simulink model "tennode_3"  (R2018b)
settings: Solver=ode3  StartTime=0.0  StopTime=5  FixedStep=Ts  RelTol=1e-3
values from neighbouring files (symbols this model uses):
  BESS_mode = 0    [load_vars.m]
  line1 = line1_length*R1    (= 0.01273)    [load_vars.m]
  line10 = line10_length*R1    (= 0.01273)    [load_vars.m]
  LINE10_en = 1    [load_vars.m]
  line11 = line11_length*R1    (= 0.01273)    [load_vars.m]
  LINE11_en = 1    [load_vars.m]
  line12 = line12_length*R1    (= 0.02546)    [load_vars.m]
  LINE12_en = 1    [load_vars.m]
  line13 = line13_length*R1    (= 0.015276)    [load_vars.m]
  LINE13_en = 1    [load_vars.m]
  line14 = line14_length*R1    (= 0.019095)    [load_vars.m]
  LINE14_en = 1    [load_vars.m]
  line15 = line15_length*R1    (= 0.014003)    [load_vars.m]
  LINE15_en = 1    [load_vars.m]
  line16 = line16_length*R1    (= 0.034371)    [load_vars.m]
  LINE16_en = 1    [load_vars.m]
  line17 = line17_length*R1    (= 0.017822)    [load_vars.m]
  LINE17_en = 1    [load_vars.m]
  LINE1_en = 1    [load_vars.m]
  line2 = line2_length*R1    (= 0.02546)    [load_vars.m]
  LINE2_en = 1    [load_vars.m]
  line3 = line3_length*R1    (= 0.015276)    [load_vars.m]
  LINE3_en = 1    [load_vars.m]
  line4 = line4_length*R1    (= 0.019095)    [load_vars.m]
  LINE4_en = 1    [load_vars.m]
  line5 = line5_length*R1    (= 0.014003)    [load_vars.m]
  LINE5_en = 1    [load_vars.m]
  line6 = line6_length*R1    (= 0.01273)    [load_vars.m]
  LINE6_en = 1    [load_vars.m]
  line7 = line7_length*R1    (= 0.03819)    [load_vars.m]
  LINE7_en = 1    [load_vars.m]
  line8 = line8_length*R1    (= 0.01273)    [load_vars.m]
  LINE8_en = 1    [load_vars.m]
  line9 = line9_length*R1    (= 0.01273)    [load_vars.m]
  LINE9_en = 1    [load_vars.m]
  t_contingency = 1    [load_vars.m]
  Ts = 0.0001    [load_vars.m]
  uDemand1 = 20e3    (= 20000)    [load_vars.m]
  uDemand10 = 20e3    (= 20000)    [load_vars.m]
  uDemand2 = 20e3    (= 20000)    [load_vars.m]
  uDemand3 = 20e3    (= 20000)    [load_vars.m]
  uDemand4 = 20e3    (= 20000)    [load_vars.m]
  uDemand5 = 20e3    (= 20000)    [load_vars.m]
  uDemand6 = 20e3    (= 20000)    [load_vars.m]
  uDemand7 = 20e3    (= 20000)    [load_vars.m]
  uDemand8 = 20e3    (= 20000)    [load_vars.m]
  uDemand9 = 20e3    (= 20000)    [load_vars.m]
undefined symbols (not defined in the file or in its folder): DER10_BESS_en, DER1_BESS_en, DER2_BESS_en, DER3_BESS_en, DER4_BESS_en, DER5_BESS_en, DER6_BESS_en, DER7_BESS_en, DER8_BESS_en, DER9_BESS_en, DR_capacity_1, DR_capacity_10, DR_capacity_2, DR_capacity_3, DR_capacity_4, DR_capacity_5, DR_capacity_6, DR_capacity_7, DR_capacity_8, DR_capacity_9, P_set1, P_set10, P_set2, P_set3, P_set4, P_set5, P_set6, P_set7, P_set8, P_set9, PV_capacity_1, PV_capacity_10, PV_capacity_2, PV_capacity_3, PV_capacity_4, PV_capacity_5, PV_capacity_6, PV_capacity_7, PV_capacity_8, PV_capacity_9, PV_en_1, PV_en_10, PV_en_2, PV_en_3, PV_en_4, PV_en_5, PV_en_6, PV_en_7, PV_en_8, PV_en_9
libraries: powerlib x232, simulink x66, powerlib_meascontrol x23, sps_avr x1, spsDieselMotorModel x1
(part 5 of 7)

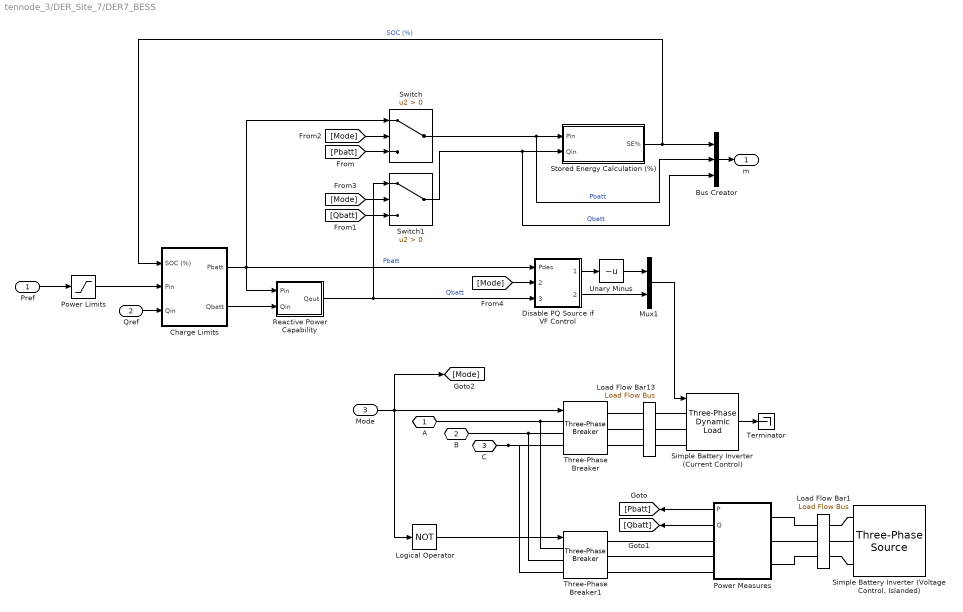
== system tennode_3/DER_Site_7/DER7_BESS ==
  Pref : Inport
  Qref : Inport  Port=2
  Mode : Inport  Port=3
  Bus Creator : BusCreator  Inputs=3
  Charge Limits : Subsystem
  Disable PQ Source if VF Control : Subsystem
  Load Flow Bar1 : powerlib/Measurements/Load Flow Bus  LConnTagsString=a|b|c  RConnTagsString=a|b|c  Phases=ABC  Connectors=on both sides  ID=5  Vbase=400/sqrt(3)  Vref=[1.0 1.0 1.0]  Vangle=[0 -120 120]  VLF=0.9823  VLFb=1.055  VLFc=0.9746  angleLF=-5.476  angleLFb=-122.5  angleLFc=116
      settings: AttributesFormatString=%<ID>  SourceProductName=Simscape Power Systems
  Load Flow Bar13 : powerlib/Measurements/Load Flow Bus  LConnTagsString=a|b|c  RConnTagsString=a|b|c  Phases=ABC  Connectors=on both sides  ID=4  Vbase=400/sqrt(3)  Vref=[1.0 1.0 1.0]  Vangle=[0 -120 120]  VLF=0.9823  VLFb=1.055  VLFc=0.9746  angleLF=-5.476  angleLFb=-122.5  angleLFc=116
      settings: AttributesFormatString=%<ID>  SourceProductName=Simscape Power Systems
  Logical Operator : Logic  Operator=NOT  AllPortsSameDT=off  OutDataTypeStr=boolean
  Mux1 : Mux  Inputs=2
  Power Limits : Saturate  UpperLimit=Pnom  LowerLimit=-Pnom
  Power Measures : Subsystem  VariantControlMode=Label  Variant=on  LabelModeActiveChoice=EMT
  Reactive Power Capability : Subsystem
  Simple Battery Inverter (Current Control) : powerlib/Elements/Three-Phase Dynamic Load  NominalVoltage=[Vn Fn]  ActiveReactivePowers=[-5000 -3.38813e-13]  PositiveSequence=[0.999844 -0.0038635]  ExternalControl=on  NpNq=[1.3 2]  TimeConstants="[0  0  0  0]"  MinimumVoltage=0.7  Tfilter=1e-2  LoadFlowParameters=[4,0,0,0,0]
      settings: SourceProductName=Simscape Electrical  SourceProductBaseCode=PS
  "Simple Battery Inverter (Voltage Control, Islanded)" : powerlib/Electrical Sources/Three-Phase Source  InternalConnection=Yg  VoltagePhases=off  Voltage=Vn  PhaseAngle=0  Voltage_phases=[25e3 25e3 25e3]/sqrt(3)  PhaseAngles_phases=[0 -120 +120]  Frequency=Fn  NonIdealSource=off  SpecifyImpedance=off  Resistance=0.8929  Inductance=16.58e-3  ShortCircuitLevel=100e6  BaseVoltage=25e3  XRratio=7  BusType=swing  Pref=10e3  Qref=0  Prefabc=[10e3, 10e3, 10e3]  Qrefabc=[0, 0, 0]  Qmin=-inf  Qmax=inf
      settings: SourceProductName=Simscape Electrical
  Stored Energy Calculation (%) : Subsystem
  Switch : Switch  Criteria=u2 > Threshold
  Switch1 : Switch  Criteria=u2 > Threshold
  Terminator : Terminator
  Three-Phase Breaker : powerlib/Elements/Three-Phase Breaker  InitialState=closed  SwitchA=on  SwitchB=on  SwitchC=on  SwitchTimes="[1/60  5/60]"  External=on  BreakerResistance=0.01  SnubberResistance=1e6  SnubberCapacitance=inf  Measurements=None
      settings: SourceProductName=Simscape Electrical
  Three-Phase Breaker1 : powerlib/Elements/Three-Phase Breaker  InitialState=open  SwitchA=on  SwitchB=on  SwitchC=on  SwitchTimes="[1/60  5/60]"  External=on  BreakerResistance=0.01  SnubberResistance=1e6  SnubberCapacitance=inf  Measurements=None
      settings: SourceProductName=Simscape Electrical
  Unary Minus : UnaryMinus
  A : PMIOPort  Side=Right
  B : PMIOPort  Port=2  Side=Right
  C : PMIOPort  Port=3  Side=Right
  m : Outport
  wires:
  Disable PQ Source if VF Control/2(Qbatt) -> Mux1/2
  Disable PQ Source if VF Control/1(Pbatt) -> Unary Minus/1
  Reactive Power Capability/1(Qout) -> Switch1/1, Disable PQ Source if VF Control/3(Qdes)  "Qbatt"
  [Mode] -> Disable PQ Source if VF Control/2(Mode)
  Charge Limits/1(Pbatt) -> Disable PQ Source if VF Control/1(Pdes), Reactive Power Capability/1(Pin), Switch/1  "Pbatt"
  [Pbatt] -> Switch/3
  [Qbatt] -> Switch1/3
  [Mode] -> Switch1/2
  [Mode] -> Switch/2
  Switch1/1 -> Stored Energy Calculation (%)/2(Qin), Bus Creator/3  "Qbatt"
  Switch/1 -> Stored Energy Calculation (%)/1(Pin), Bus Creator/2  "Pbatt"
  Power Measures/2(Q) -> [Qbatt]
  Power Measures/1(P) -> [Pbatt]
  Mode/1 -> Three-Phase Breaker/1, Logical Operator/1, [Mode]
  Logical Operator/1 -> Three-Phase Breaker1/1
  Unary Minus/1 -> Mux1/1
  Mux1/1 -> Simple Battery Inverter (Current Control)/1
  Simple Battery Inverter (Current Control)/1 -> Terminator/1
  Pref/1 -> Power Limits/1
  Bus Creator/1 -> m/1
  Stored Energy Calculation (%)/1(SE%) -> Charge Limits/1(SOC (%)), Bus Creator/1  "SOC (%)"
  Power Limits/1 -> Charge Limits/2(Pin)
  Qref/1 -> Charge Limits/3(Qin)
  Charge Limits/2(Qbatt) -> Reactive Power Capability/2(Qin)
  connections:
  Power Measures/RConn3 -- Three-Phase Breaker1/RConn3
  Power Measures/RConn2 -- Three-Phase Breaker1/RConn2
  Power Measures/RConn1 -- Three-Phase Breaker1/RConn1
  Three-Phase Breaker1/LConn1 -- A/RConn1 -- Three-Phase Breaker/LConn1
  Three-Phase Breaker1/LConn2 -- B/RConn1 -- Three-Phase Breaker/LConn2
  C/RConn1 -- Three-Phase Breaker1/LConn3 -- Three-Phase Breaker/LConn3
  Load Flow Bar13/RConn1 -- Three-Phase Breaker/RConn1
  Load Flow Bar13/RConn2 -- Three-Phase Breaker/RConn2
  Load Flow Bar13/RConn3 -- Three-Phase Breaker/RConn3
  Load Flow Bar13/LConn1 -- Simple Battery Inverter (Current Control)/LConn1
  Load Flow Bar13/LConn2 -- Simple Battery Inverter (Current Control)/LConn2
  Load Flow Bar13/LConn3 -- Simple Battery Inverter (Current Control)/LConn3
  "Simple Battery Inverter (Voltage Control, Islanded)"/RConn2 -- Load Flow Bar1/LConn2
  Load Flow Bar1/LConn3 -- "Simple Battery Inverter (Voltage Control, Islanded)"/RConn3
  Load Flow Bar1/LConn1 -- "Simple Battery Inverter (Voltage Control, Islanded)"/RConn1
  Power Measures/LConn1 -- Load Flow Bar1/RConn1
  Power Measures/LConn2 -- Load Flow Bar1/RConn2
  Power Measures/LConn3 -- Load Flow Bar1/RConn3

== system tennode_3/DER_Site_7/DER7_PV  ==
  P : Inport
  Bus Selector : BusSelector  OutputSignals=Active power P (W)
  Constant11 : Constant  Value=0
  Mux1 : Mux  Inputs=2
  Simple Solar Inverter : powerlib/Elements/Three-Phase Dynamic Load  NominalVoltage=[Vn Fn]  ActiveReactivePowers=[-4000 -3.38813e-13]  PositiveSequence=[0.999844 -0.0038635]  ExternalControl=on  NpNq=[1.3 2]  TimeConstants="[0  0  0  0]"  MinimumVoltage=0.7  Tfilter=1e-2  LoadFlowParameters=[4,0,0,0,0]
      settings: SourceProductName=Simscape Electrical  SourceProductBaseCode=PS
  Unary Minus : UnaryMinus
  Unary Minus1 : UnaryMinus
  A : PMIOPort  Side=Right
  B : PMIOPort  Port=2  Side=Right
  C : PMIOPort  Port=3  Side=Right
  m : Outport
  wires:
  P/1 -> Unary Minus/1
  Unary Minus/1 -> Mux1/1
  Mux1/1 -> Simple Solar Inverter/1
  Constant11/1 -> Mux1/2
  Simple Solar Inverter/1 -> Bus Selector/1
  Bus Selector/1 -> Unary Minus1/1  "<Active power P (W)>"
  Unary Minus1/1 -> m/1
  connections:
  Simple Solar Inverter/LConn2 -- B/RConn1
  Simple Solar Inverter/LConn3 -- C/RConn1
  Simple Solar Inverter/LConn1 -- A/RConn1

== system tennode_3/DER_Site_7/Site Load ==
  Load : Inport
  Dynamic Load Control : Subsystem
  Simple Three-Phase Load : powerlib/Elements/Three-Phase Dynamic Load  NominalVoltage=[Vn Fn]  ActiveReactivePowers=[200000 45883.1]  PositiveSequence=[0.999844 -0.0038635]  ExternalControl=on  NpNq=[1.3 2]  TimeConstants="[0  0  0  0]"  MinimumVoltage=0.7  Tfilter=1e-2  LoadFlowParameters=[4,0,0,0,0]
      settings: SourceProductName=Simscape Electrical  SourceProductBaseCode=PS
  A : PMIOPort  Side=Right
  B : PMIOPort  Port=2  Side=Right
  C : PMIOPort  Port=3  Side=Right
  m : Outport
  wires:
  Load/1 -> Dynamic Load Control/1(P0)
  Dynamic Load Control/1(PQ) -> Simple Three-Phase Load/1
  Simple Three-Phase Load/1 -> m/1
  connections:
  Simple Three-Phase Load/LConn1 -- A/RConn1
  Simple Three-Phase Load/LConn3 -- C/RConn1
  Simple Three-Phase Load/LConn2 -- B/RConn1

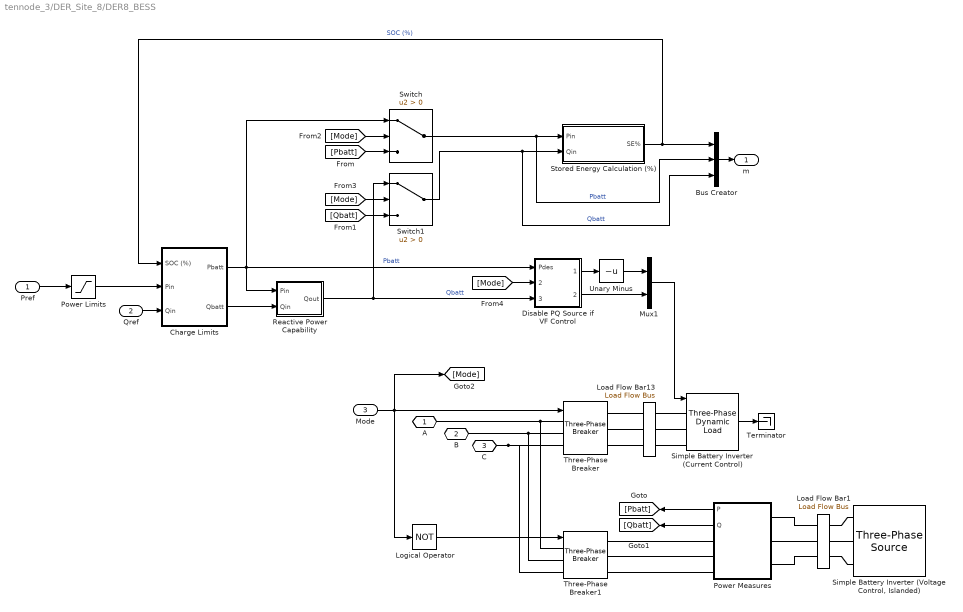
== system tennode_3/DER_Site_8/DER8_BESS ==
  Pref : Inport
  Qref : Inport  Port=2
  Mode : Inport  Port=3
  Bus Creator : BusCreator  Inputs=3
  Charge Limits : Subsystem
  Disable PQ Source if VF Control : Subsystem
  Load Flow Bar1 : powerlib/Measurements/Load Flow Bus  LConnTagsString=a|b|c  RConnTagsString=a|b|c  Phases=ABC  Connectors=on both sides  ID=5  Vbase=400/sqrt(3)  Vref=[1.0 1.0 1.0]  Vangle=[0 -120 120]  VLF=0.9823  VLFb=1.055  VLFc=0.9746  angleLF=-5.476  angleLFb=-122.5  angleLFc=116
      settings: AttributesFormatString=%<ID>  SourceProductName=Simscape Power Systems
  Load Flow Bar13 : powerlib/Measurements/Load Flow Bus  LConnTagsString=a|b|c  RConnTagsString=a|b|c  Phases=ABC  Connectors=on both sides  ID=4  Vbase=400/sqrt(3)  Vref=[1.0 1.0 1.0]  Vangle=[0 -120 120]  VLF=0.9823  VLFb=1.055  VLFc=0.9746  angleLF=-5.476  angleLFb=-122.5  angleLFc=116
      settings: AttributesFormatString=%<ID>  SourceProductName=Simscape Power Systems
  Logical Operator : Logic  Operator=NOT  AllPortsSameDT=off  OutDataTypeStr=boolean
  Mux1 : Mux  Inputs=2
  Power Limits : Saturate  UpperLimit=Pnom  LowerLimit=-Pnom
  Power Measures : Subsystem  VariantControlMode=Label  Variant=on  LabelModeActiveChoice=EMT
  Reactive Power Capability : Subsystem
  Simple Battery Inverter (Current Control) : powerlib/Elements/Three-Phase Dynamic Load  NominalVoltage=[Vn Fn]  ActiveReactivePowers=[-5000 -3.38813e-13]  PositiveSequence=[0.999844 -0.0038635]  ExternalControl=on  NpNq=[1.3 2]  TimeConstants="[0  0  0  0]"  MinimumVoltage=0.7  Tfilter=1e-2  LoadFlowParameters=[4,0,0,0,0]
      settings: SourceProductName=Simscape Electrical  SourceProductBaseCode=PS
  "Simple Battery Inverter (Voltage Control, Islanded)" : powerlib/Electrical Sources/Three-Phase Source  InternalConnection=Yg  VoltagePhases=off  Voltage=Vn  PhaseAngle=0  Voltage_phases=[25e3 25e3 25e3]/sqrt(3)  PhaseAngles_phases=[0 -120 +120]  Frequency=Fn  NonIdealSource=off  SpecifyImpedance=off  Resistance=0.8929  Inductance=16.58e-3  ShortCircuitLevel=100e6  BaseVoltage=25e3  XRratio=7  BusType=swing  Pref=10e3  Qref=0  Prefabc=[10e3, 10e3, 10e3]  Qrefabc=[0, 0, 0]  Qmin=-inf  Qmax=inf
      settings: SourceProductName=Simscape Electrical
  Stored Energy Calculation (%) : Subsystem
  Switch : Switch  Criteria=u2 > Threshold
  Switch1 : Switch  Criteria=u2 > Threshold
  Terminator : Terminator
  Three-Phase Breaker : powerlib/Elements/Three-Phase Breaker  InitialState=closed  SwitchA=on  SwitchB=on  SwitchC=on  SwitchTimes="[1/60  5/60]"  External=on  BreakerResistance=0.01  SnubberResistance=1e6  SnubberCapacitance=inf  Measurements=None
      settings: SourceProductName=Simscape Electrical
  Three-Phase Breaker1 : powerlib/Elements/Three-Phase Breaker  InitialState=open  SwitchA=on  SwitchB=on  SwitchC=on  SwitchTimes="[1/60  5/60]"  External=on  BreakerResistance=0.01  SnubberResistance=1e6  SnubberCapacitance=inf  Measurements=None
      settings: SourceProductName=Simscape Electrical
  Unary Minus : UnaryMinus
  A : PMIOPort  Side=Right
  B : PMIOPort  Port=2  Side=Right
  C : PMIOPort  Port=3  Side=Right
  m : Outport
  wires:
  Disable PQ Source if VF Control/2(Qbatt) -> Mux1/2
  Disable PQ Source if VF Control/1(Pbatt) -> Unary Minus/1
  Reactive Power Capability/1(Qout) -> Switch1/1, Disable PQ Source if VF Control/3(Qdes)  "Qbatt"
  [Mode] -> Disable PQ Source if VF Control/2(Mode)
  Charge Limits/1(Pbatt) -> Disable PQ Source if VF Control/1(Pdes), Reactive Power Capability/1(Pin), Switch/1  "Pbatt"
  [Pbatt] -> Switch/3
  [Qbatt] -> Switch1/3
  [Mode] -> Switch1/2
  [Mode] -> Switch/2
  Switch1/1 -> Stored Energy Calculation (%)/2(Qin), Bus Creator/3  "Qbatt"
  Switch/1 -> Stored Energy Calculation (%)/1(Pin), Bus Creator/2  "Pbatt"
  Power Measures/2(Q) -> [Qbatt]
  Power Measures/1(P) -> [Pbatt]
  Mode/1 -> Three-Phase Breaker/1, Logical Operator/1, [Mode]
  Logical Operator/1 -> Three-Phase Breaker1/1
  Unary Minus/1 -> Mux1/1
  Mux1/1 -> Simple Battery Inverter (Current Control)/1
  Simple Battery Inverter (Current Control)/1 -> Terminator/1
  Pref/1 -> Power Limits/1
  Bus Creator/1 -> m/1
  Stored Energy Calculation (%)/1(SE%) -> Charge Limits/1(SOC (%)), Bus Creator/1  "SOC (%)"
  Power Limits/1 -> Charge Limits/2(Pin)
  Qref/1 -> Charge Limits/3(Qin)
  Charge Limits/2(Qbatt) -> Reactive Power Capability/2(Qin)
  connections:
  Power Measures/RConn3 -- Three-Phase Breaker1/RConn3
  Power Measures/RConn2 -- Three-Phase Breaker1/RConn2
  Power Measures/RConn1 -- Three-Phase Breaker1/RConn1
  Three-Phase Breaker1/LConn1 -- A/RConn1 -- Three-Phase Breaker/LConn1
  Three-Phase Breaker1/LConn2 -- B/RConn1 -- Three-Phase Breaker/LConn2
  C/RConn1 -- Three-Phase Breaker1/LConn3 -- Three-Phase Breaker/LConn3
  Load Flow Bar13/RConn1 -- Three-Phase Breaker/RConn1
  Load Flow Bar13/RConn2 -- Three-Phase Breaker/RConn2
  Load Flow Bar13/RConn3 -- Three-Phase Breaker/RConn3
  Load Flow Bar13/LConn1 -- Simple Battery Inverter (Current Control)/LConn1
  Load Flow Bar13/LConn2 -- Simple Battery Inverter (Current Control)/LConn2
  Load Flow Bar13/LConn3 -- Simple Battery Inverter (Current Control)/LConn3
  "Simple Battery Inverter (Voltage Control, Islanded)"/RConn2 -- Load Flow Bar1/LConn2
  Load Flow Bar1/LConn3 -- "Simple Battery Inverter (Voltage Control, Islanded)"/RConn3
  Load Flow Bar1/LConn1 -- "Simple Battery Inverter (Voltage Control, Islanded)"/RConn1
  Power Measures/LConn1 -- Load Flow Bar1/RConn1
  Power Measures/LConn2 -- Load Flow Bar1/RConn2
  Power Measures/LConn3 -- Load Flow Bar1/RConn3

== system tennode_3/DER_Site_8/DER8_PV  ==
  P : Inport
  Bus Selector : BusSelector  OutputSignals=Active power P (W)
  Constant11 : Constant  Value=0
  Mux1 : Mux  Inputs=2
  Simple Solar Inverter : powerlib/Elements/Three-Phase Dynamic Load  NominalVoltage=[Vn Fn]  ActiveReactivePowers=[-4000 -3.38813e-13]  PositiveSequence=[0.999844 -0.0038635]  ExternalControl=on  NpNq=[1.3 2]  TimeConstants="[0  0  0  0]"  MinimumVoltage=0.7  Tfilter=1e-2  LoadFlowParameters=[4,0,0,0,0]
      settings: SourceProductName=Simscape Electrical  SourceProductBaseCode=PS
  Unary Minus : UnaryMinus
  Unary Minus1 : UnaryMinus
  A : PMIOPort  Side=Right
  B : PMIOPort  Port=2  Side=Right
  C : PMIOPort  Port=3  Side=Right
  m : Outport
  wires:
  P/1 -> Unary Minus/1
  Unary Minus/1 -> Mux1/1
  Mux1/1 -> Simple Solar Inverter/1
  Constant11/1 -> Mux1/2
  Simple Solar Inverter/1 -> Bus Selector/1
  Bus Selector/1 -> Unary Minus1/1  "<Active power P (W)>"
  Unary Minus1/1 -> m/1
  connections:
  Simple Solar Inverter/LConn2 -- B/RConn1
  Simple Solar Inverter/LConn3 -- C/RConn1
  Simple Solar Inverter/LConn1 -- A/RConn1

== system tennode_3/DER_Site_8/Site Load ==
  Load : Inport
  Dynamic Load Control : Subsystem
  Simple Three-Phase Load : powerlib/Elements/Three-Phase Dynamic Load  NominalVoltage=[Vn Fn]  ActiveReactivePowers=[200000 45883.1]  PositiveSequence=[0.999844 -0.0038635]  ExternalControl=on  NpNq=[1.3 2]  TimeConstants="[0  0  0  0]"  MinimumVoltage=0.7  Tfilter=1e-2  LoadFlowParameters=[4,0,0,0,0]
      settings: SourceProductName=Simscape Electrical  SourceProductBaseCode=PS
  A : PMIOPort  Side=Right
  B : PMIOPort  Port=2  Side=Right
  C : PMIOPort  Port=3  Side=Right
  m : Outport
  wires:
  Load/1 -> Dynamic Load Control/1(P0)
  Dynamic Load Control/1(PQ) -> Simple Three-Phase Load/1
  Simple Three-Phase Load/1 -> m/1
  connections:
  Simple Three-Phase Load/LConn1 -- A/RConn1
  Simple Three-Phase Load/LConn3 -- C/RConn1
  Simple Three-Phase Load/LConn2 -- B/RConn1

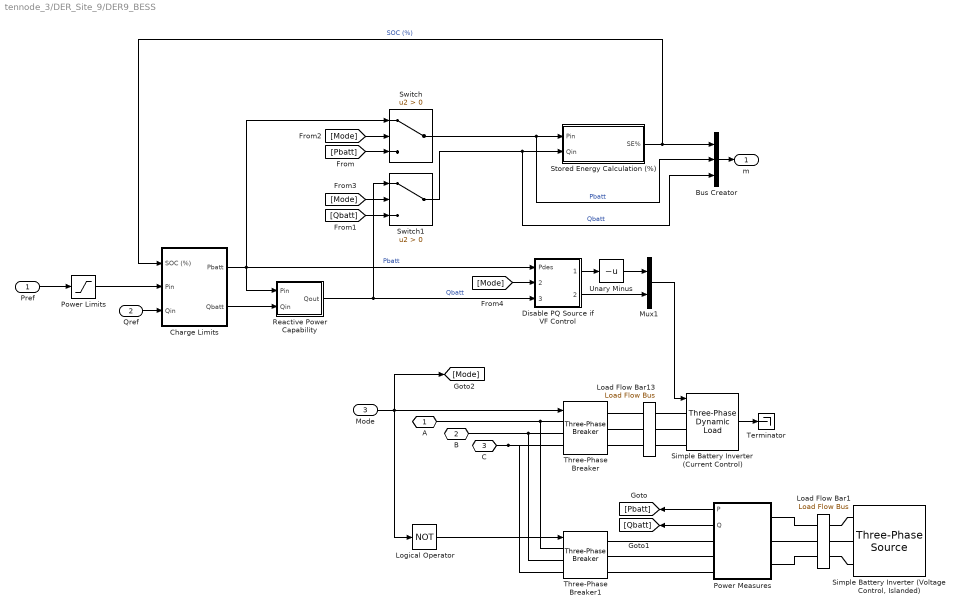
== system tennode_3/DER_Site_9/DER9_BESS ==
  Pref : Inport
  Qref : Inport  Port=2
  Mode : Inport  Port=3
  Bus Creator : BusCreator  Inputs=3
  Charge Limits : Subsystem
  Disable PQ Source if VF Control : Subsystem
  Load Flow Bar1 : powerlib/Measurements/Load Flow Bus  LConnTagsString=a|b|c  RConnTagsString=a|b|c  Phases=ABC  Connectors=on both sides  ID=5  Vbase=400/sqrt(3)  Vref=[1.0 1.0 1.0]  Vangle=[0 -120 120]  VLF=0.9823  VLFb=1.055  VLFc=0.9746  angleLF=-5.476  angleLFb=-122.5  angleLFc=116
      settings: AttributesFormatString=%<ID>  SourceProductName=Simscape Power Systems
  Load Flow Bar13 : powerlib/Measurements/Load Flow Bus  LConnTagsString=a|b|c  RConnTagsString=a|b|c  Phases=ABC  Connectors=on both sides  ID=4  Vbase=400/sqrt(3)  Vref=[1.0 1.0 1.0]  Vangle=[0 -120 120]  VLF=0.9823  VLFb=1.055  VLFc=0.9746  angleLF=-5.476  angleLFb=-122.5  angleLFc=116
      settings: AttributesFormatString=%<ID>  SourceProductName=Simscape Power Systems
  Logical Operator : Logic  Operator=NOT  AllPortsSameDT=off  OutDataTypeStr=boolean
  Mux1 : Mux  Inputs=2
  Power Limits : Saturate  UpperLimit=Pnom  LowerLimit=-Pnom
  Power Measures : Subsystem  VariantControlMode=Label  Variant=on  LabelModeActiveChoice=EMT
  Reactive Power Capability : Subsystem
  Simple Battery Inverter (Current Control) : powerlib/Elements/Three-Phase Dynamic Load  NominalVoltage=[Vn Fn]  ActiveReactivePowers=[-5000 -3.38813e-13]  PositiveSequence=[0.999844 -0.0038635]  ExternalControl=on  NpNq=[1.3 2]  TimeConstants="[0  0  0  0]"  MinimumVoltage=0.7  Tfilter=1e-2  LoadFlowParameters=[4,0,0,0,0]
      settings: SourceProductName=Simscape Electrical  SourceProductBaseCode=PS
  "Simple Battery Inverter (Voltage Control, Islanded)" : powerlib/Electrical Sources/Three-Phase Source  InternalConnection=Yg  VoltagePhases=off  Voltage=Vn  PhaseAngle=0  Voltage_phases=[25e3 25e3 25e3]/sqrt(3)  PhaseAngles_phases=[0 -120 +120]  Frequency=Fn  NonIdealSource=off  SpecifyImpedance=off  Resistance=0.8929  Inductance=16.58e-3  ShortCircuitLevel=100e6  BaseVoltage=25e3  XRratio=7  BusType=swing  Pref=10e3  Qref=0  Prefabc=[10e3, 10e3, 10e3]  Qrefabc=[0, 0, 0]  Qmin=-inf  Qmax=inf
      settings: SourceProductName=Simscape Electrical
  Stored Energy Calculation (%) : Subsystem
  Switch : Switch  Criteria=u2 > Threshold
  Switch1 : Switch  Criteria=u2 > Threshold
  Terminator : Terminator
  Three-Phase Breaker : powerlib/Elements/Three-Phase Breaker  InitialState=closed  SwitchA=on  SwitchB=on  SwitchC=on  SwitchTimes="[1/60  5/60]"  External=on  BreakerResistance=0.01  SnubberResistance=1e6  SnubberCapacitance=inf  Measurements=None
      settings: SourceProductName=Simscape Electrical
  Three-Phase Breaker1 : powerlib/Elements/Three-Phase Breaker  InitialState=open  SwitchA=on  SwitchB=on  SwitchC=on  SwitchTimes="[1/60  5/60]"  External=on  BreakerResistance=0.01  SnubberResistance=1e6  SnubberCapacitance=inf  Measurements=None
      settings: SourceProductName=Simscape Electrical
  Unary Minus : UnaryMinus
  A : PMIOPort  Side=Right
  B : PMIOPort  Port=2  Side=Right
  C : PMIOPort  Port=3  Side=Right
  m : Outport
  wires:
  Disable PQ Source if VF Control/2(Qbatt) -> Mux1/2
  Disable PQ Source if VF Control/1(Pbatt) -> Unary Minus/1
  Reactive Power Capability/1(Qout) -> Switch1/1, Disable PQ Source if VF Control/3(Qdes)  "Qbatt"
  [Mode] -> Disable PQ Source if VF Control/2(Mode)
  Charge Limits/1(Pbatt) -> Disable PQ Source if VF Control/1(Pdes), Reactive Power Capability/1(Pin), Switch/1  "Pbatt"
  [Pbatt] -> Switch/3
  [Qbatt] -> Switch1/3
  [Mode] -> Switch1/2
  [Mode] -> Switch/2
  Switch1/1 -> Stored Energy Calculation (%)/2(Qin), Bus Creator/3  "Qbatt"
  Switch/1 -> Stored Energy Calculation (%)/1(Pin), Bus Creator/2  "Pbatt"
  Power Measures/2(Q) -> [Qbatt]
  Power Measures/1(P) -> [Pbatt]
  Mode/1 -> Three-Phase Breaker/1, Logical Operator/1, [Mode]
  Logical Operator/1 -> Three-Phase Breaker1/1
  Unary Minus/1 -> Mux1/1
  Mux1/1 -> Simple Battery Inverter (Current Control)/1
  Simple Battery Inverter (Current Control)/1 -> Terminator/1
  Pref/1 -> Power Limits/1
  Bus Creator/1 -> m/1
  Stored Energy Calculation (%)/1(SE%) -> Charge Limits/1(SOC (%)), Bus Creator/1  "SOC (%)"
  Power Limits/1 -> Charge Limits/2(Pin)
  Qref/1 -> Charge Limits/3(Qin)
  Charge Limits/2(Qbatt) -> Reactive Power Capability/2(Qin)
  connections:
  Power Measures/RConn3 -- Three-Phase Breaker1/RConn3
  Power Measures/RConn2 -- Three-Phase Breaker1/RConn2
  Power Measures/RConn1 -- Three-Phase Breaker1/RConn1
  Three-Phase Breaker1/LConn1 -- A/RConn1 -- Three-Phase Breaker/LConn1
  Three-Phase Breaker1/LConn2 -- B/RConn1 -- Three-Phase Breaker/LConn2
  C/RConn1 -- Three-Phase Breaker1/LConn3 -- Three-Phase Breaker/LConn3
  Load Flow Bar13/RConn1 -- Three-Phase Breaker/RConn1
  Load Flow Bar13/RConn2 -- Three-Phase Breaker/RConn2
  Load Flow Bar13/RConn3 -- Three-Phase Breaker/RConn3
  Load Flow Bar13/LConn1 -- Simple Battery Inverter (Current Control)/LConn1
  Load Flow Bar13/LConn2 -- Simple Battery Inverter (Current Control)/LConn2
  Load Flow Bar13/LConn3 -- Simple Battery Inverter (Current Control)/LConn3
  "Simple Battery Inverter (Voltage Control, Islanded)"/RConn2 -- Load Flow Bar1/LConn2
  Load Flow Bar1/LConn3 -- "Simple Battery Inverter (Voltage Control, Islanded)"/RConn3
  Load Flow Bar1/LConn1 -- "Simple Battery Inverter (Voltage Control, Islanded)"/RConn1
  Power Measures/LConn1 -- Load Flow Bar1/RConn1
  Power Measures/LConn2 -- Load Flow Bar1/RConn2
  Power Measures/LConn3 -- Load Flow Bar1/RConn3

== system tennode_3/DER_Site_9/DER9_PV  ==
  P : Inport
  Bus Selector : BusSelector  OutputSignals=Active power P (W)
  Constant11 : Constant  Value=0
  Mux1 : Mux  Inputs=2
  Simple Solar Inverter : powerlib/Elements/Three-Phase Dynamic Load  NominalVoltage=[Vn Fn]  ActiveReactivePowers=[-4000 -3.38813e-13]  PositiveSequence=[0.999844 -0.0038635]  ExternalControl=on  NpNq=[1.3 2]  TimeConstants="[0  0  0  0]"  MinimumVoltage=0.7  Tfilter=1e-2  LoadFlowParameters=[4,0,0,0,0]
      settings: SourceProductName=Simscape Electrical  SourceProductBaseCode=PS
  Unary Minus : UnaryMinus
  Unary Minus1 : UnaryMinus
  A : PMIOPort  Side=Right
  B : PMIOPort  Port=2  Side=Right
  C : PMIOPort  Port=3  Side=Right
  m : Outport
  wires:
  P/1 -> Unary Minus/1
  Unary Minus/1 -> Mux1/1
  Mux1/1 -> Simple Solar Inverter/1
  Constant11/1 -> Mux1/2
  Simple Solar Inverter/1 -> Bus Selector/1
  Bus Selector/1 -> Unary Minus1/1  "<Active power P (W)>"
  Unary Minus1/1 -> m/1
  connections:
  Simple Solar Inverter/LConn2 -- B/RConn1
  Simple Solar Inverter/LConn3 -- C/RConn1
  Simple Solar Inverter/LConn1 -- A/RConn1

== system tennode_3/DER_Site_9/Site Load ==
  Load : Inport
  Dynamic Load Control : Subsystem
  Simple Three-Phase Load : powerlib/Elements/Three-Phase Dynamic Load  NominalVoltage=[Vn Fn]  ActiveReactivePowers=[200000 45883.1]  PositiveSequence=[0.999844 -0.0038635]  ExternalControl=on  NpNq=[1.3 2]  TimeConstants="[0  0  0  0]"  MinimumVoltage=0.7  Tfilter=1e-2  LoadFlowParameters=[4,0,0,0,0]
      settings: SourceProductName=Simscape Electrical  SourceProductBaseCode=PS
  A : PMIOPort  Side=Right
  B : PMIOPort  Port=2  Side=Right
  C : PMIOPort  Port=3  Side=Right
  m : Outport
  wires:
  Load/1 -> Dynamic Load Control/1(P0)
  Dynamic Load Control/1(PQ) -> Simple Three-Phase Load/1
  Simple Three-Phase Load/1 -> m/1
  connections:
  Simple Three-Phase Load/LConn1 -- A/RConn1
  Simple Three-Phase Load/LConn3 -- C/RConn1
  Simple Three-Phase Load/LConn2 -- B/RConn1

== system tennode_3/Frequency Measure/Diesel Generator ==
  wref (pu) : Inport
  Vref (pu) : Inport  Port=2
  AC1A Excitation System : sps_avr/AC1A Excitation System  Tr=20e-3  KaTa=[400 0.02]  VAminmax=[-14.5 14.5]  VRminmax=[-5.43 6.03]  KfTf=[0.03 1.0]  TbTc=[0 0]  KeTe=[1.0 0.80]  Ve12=[4.18 3.14]  SeVe12=[0.10 0.03]  Kd=0.38  Kc=0.20  v0=[0.99984 1.0013]  TsBlock=0
      settings: SourceProductName=Simscape Electrical  SourceProductBaseCode=PS
  Diesel Engine Governor : spsDieselMotorModel/Diesel Engine Governor  K=29  Tr=[0.01 0.02 0.2]  Ta=[0.25 0.009 0.0384]  Tlim=[0 1.1]  Td=0.024  Pm0=0.050008
  Generator Measures : Subsystem
  Ground : Ground
  Selected Measurements : Subsystem
  Shunt : powerlib/Elements/Three-Phase Parallel RLC Load  Commented=on  LConnTagsString=A|B|C  Configuration=Y (grounded)  NominalVoltage=Vn  Vabc=[1e3 1e3 1e3]  Vabcp=[1e3 1e3 1e3]  NominalFrequency=Fn  UnbalancedPower=off  ActivePower=Pn*0.05  InductivePower=0  CapacitivePower=0  Pabc=[10e3 9e3 11e3]  QLabc=[100 90 110]  QCabc=[100 90 110]  Pabcp=[10e3 9e3 11e3]  QLabcp=[100 90 110]  QCabcp=[100 90 110]  Measurements=None  LoadType=constant Z
      settings: SourceProductName=Simscape Electrical
  Synchronous Machine : powerlib/Machines/Synchronous Machine pu Standard  PresetModel=No  MechanicalLoad=Mechanical power Pm  ShowDetailedParameters=on  RotorType=Salient-pole  Units=per unit standard parameters  MeasurementBus=off  NominalParameters=[ Pn Vn Fn]  Reactances1=[ 1.81, 0.3, 0.23, 1.76, 0.65, 0.25, 0.15 ]  Reactances2="[ 1.305, 0.296, 0.252, 0.474,  0.243,  0.18 ]"  dAxisTimeConstants=Open-circuit  qAxisTimeConstants=Short-circuit  TimeConstants1="[ 4.4849  0.0681  0.1  ]"  TimeConstants2=[ 8.0, 0.03, 1.0, 0.07 ]  TimeConstants3="[  4.49  0.0681  0.0513  ]"  TimeConstants4=[ 8.0, 0.03, 0.3371, 0.0295 ]  TimeConstants5=[ 1.01, 0.053, 0.1 ]  TimeConstants6=[ 1.3201, 0.023, 1.0, 0.07 ]  TimeConstants7=[0.012 0.003 0.003]  TimeConstants8=[ 1.3201, 0.0231, 0.3371, 0.0295 ]  StatorResistance=0.003  Mechanical=[3.7 0 1 ]  PolePairs=20  InitialConditions=[0 -88.646 0.0500078 0.0500078 0.0500078 -0.0038635 -120.004 119.996 1.00126]  SetSaturation=off  Saturation=[0.6404,0.7127,0.8441,0.9214,0.9956,1.082,1.19,1.316,1.457;0.7,0.7698,0.8872,0.9466,0.9969,1.046,1.1,1.151,1.201]  LoadFlowParameters=[1,0,0,0,0]  TsPowergui=0  TsBlock=-1  IterativeModel=Trapezoidal non iterative  IterativeDiscreteModel=Trapezoidal non iterative  BusType=PQ  Pref=Pn*P0  Qref=0  Qmin=-inf  Qmax=inf  PLF=0  QLF=0
      settings: SourceProductName=Simscape Electrical
  A : PMIOPort  Side=Right
  B : PMIOPort  Port=2  Side=Right
  C : PMIOPort  Port=3  Side=Right
  m : Outport
  wires:
  wref (pu)/1 -> Diesel Engine Governor/1
  Diesel Engine Governor/1 -> Synchronous Machine/1
  AC1A Excitation System/1 -> Synchronous Machine/2
  Vref (pu)/1 -> AC1A Excitation System/1
  Synchronous Machine/1 -> Generator Measures/1(m), Selected Measurements/1(m)
  Ground/1 -> AC1A Excitation System/4
  Generator Measures/3(wm) -> Diesel Engine Governor/2
  Generator Measures/2(Vt) -> AC1A Excitation System/2
  Generator Measures/1(Ifd) -> AC1A Excitation System/3
  Selected Measurements/1(sm) -> m/1
  connections:
  Shunt/LConn1 -- Synchronous Machine/RConn1 -- A/RConn1
  Synchronous Machine/RConn3 -- Shunt/LConn3 -- C/RConn1
  Synchronous Machine/RConn2 -- Shunt/LConn2 -- B/RConn1

== system tennode_3/DER_BESS1/Charge Limits/Overcharge Check ==
  SOC (%) : Inport
  Pin : Inport  Port=2
  Qin : Inport  Port=3
  Backlash : Backlash  BacklashWidth=1e-3  InitialOutput=Initial_kWh_pc  ZeroCross=off
  Compare To Constant : simulink/Logic and Bit Operations/Compare To Constant  relop=>  const=UpChrgLim  OutDataTypeStr=boolean
  Compare To Zero : simulink/Logic and Bit Operations/Compare To Zero  relop=<=  OutDataTypeStr=boolean
  Constant : Constant  Value=0
  Constant1 : Constant  Value=0
  Logical Operator : Logic  AllPortsSameDT=off  OutDataTypeStr=boolean
  Switch : Switch  Criteria=u2 ~= 0
  Switch1 : Switch  Criteria=u2 ~= 0
  Pout : Outport
  Qout : Outport  Port=2
  wires:
  Compare To Constant/1 -> Logical Operator/1
  Logical Operator/1 -> Switch1/2, Switch/2
  Constant/1 -> Switch/1
  SOC (%)/1 -> Backlash/1
  Pin/1 -> Compare To Zero/1, Switch/3
  Switch/1 -> Pout/1
  Compare To Zero/1 -> Logical Operator/2
  Qin/1 -> Switch1/3
  Constant1/1 -> Switch1/1
  Switch1/1 -> Qout/1
  Backlash/1 -> Compare To Constant/1

== system tennode_3/DER_BESS1/Charge Limits/Undercharge Check ==
  SOC (%) : Inport
  Pin : Inport  Port=2
  Qin : Inport  Port=3
  Backlash : Backlash  BacklashWidth=1e-3  InitialOutput=Initial_kWh_pc  ZeroCross=off
  Compare To Constant1 : simulink/Logic and Bit Operations/Compare To Constant  relop=<  const=LowChrgLim  OutDataTypeStr=boolean
  Compare To Zero : simulink/Logic and Bit Operations/Compare To Zero  relop=>  OutDataTypeStr=boolean
  Constant{,1..3} (4 alike) : Constant  Value=0
  Constant4 : Constant  Value=autoRecharge
  IC : InitialCondition  Value=RechargeSOC
  Logical Operator : Logic  AllPortsSameDT=off  OutDataTypeStr=boolean
  Relay : Relay  OnSwitchValue=RechargeSOC  OffSwitchValue=LowChrgLim  OnOutputValue=0  OffOutputValue=-Precharge/100*Pnom
  Switch{,1..4} (5 alike) : Switch  Criteria=u2 ~= 0
  Pout : Outport
  Qout : Outport  Port=2
  wires:
  Compare To Zero/1 -> Logical Operator/2
  Pin/1 -> Switch/3, Compare To Zero/1
  SOC (%)/1 -> Backlash/1
  Constant/1 -> Switch/1
  Logical Operator/1 -> Switch/2, Switch1/2
  Compare To Constant1/1 -> Logical Operator/1
  Constant1/1 -> Switch1/1
  Qin/1 -> Switch1/3
  Backlash/1 -> IC/1, Compare To Constant1/1
  Switch4/1 -> Switch2/1, Switch2/2, Switch3/2
  IC/1 -> Relay/1
  Switch/1 -> Switch2/3
  Switch2/1 -> Pout/1
  Switch3/1 -> Qout/1
  Switch1/1 -> Switch3/3
  Constant2/1 -> Switch3/1
  Relay/1 -> Switch4/1
  Constant3/1 -> Switch4/3
  Constant4/1 -> Switch4/2

== system tennode_3/DER_BESS1/Power Measures/EMT ==
  "Power (3ph, Instantaneous)" : powerlib_meascontrol/Measurements/Power (3ph, Instantaneous)
      settings: SourceProductName=Simscape Electrical
  Three-Phase V-I Measurement : powerlib/Measurements/Three-Phase V-I Measurement  VoltageMeasurement=phase-to-ground  SetLabelV=off  LabelV=Vabc  Vpu=off  VpuLL=off  CurrentMeasurement=yes  SetLabelI=off  LabelI=Iabc  Ipu=off  Pbase=100e6  Vbase=500e3  OutputType=Complex  PhasorSimulation=on  PSBequivalent=0
      settings: SourceProductName=Simscape Electrical
  A : PMIOPort  Side=Left
  a : PMIOPort  Port=2  Side=Right
  B : PMIOPort  Port=3  Side=Left
  b : PMIOPort  Port=4  Side=Right
  C : PMIOPort  Port=5  Side=Left
  c : PMIOPort  Port=6  Side=Right
  P : Outport
  Q : Outport  Port=2
  wires:
  "Power (3ph, Instantaneous)"/2 -> Q/1
  "Power (3ph, Instantaneous)"/1 -> P/1
  Three-Phase V-I Measurement/1 -> "Power (3ph, Instantaneous)"/1
  Three-Phase V-I Measurement/2 -> "Power (3ph, Instantaneous)"/2
  connections:
  C/RConn1 -- Three-Phase V-I Measurement/LConn3
  c/RConn1 -- Three-Phase V-I Measurement/RConn3
  Three-Phase V-I Measurement/LConn2 -- B/RConn1
  A/RConn1 -- Three-Phase V-I Measurement/LConn1
  b/RConn1 -- Three-Phase V-I Measurement/RConn2
  Three-Phase V-I Measurement/RConn1 -- a/RConn1

== system tennode_3/DER_BESS1/Power Measures/Phasor ==
  "Power (3ph, Phasor)" : powerlib_meascontrol/Measurements/Power (3ph, Phasor)
      settings: SourceProductName=Simscape Electrical  SourceProductBaseCode=PS
  Three-Phase V-I Measurement : powerlib/Measurements/Three-Phase V-I Measurement  VoltageMeasurement=phase-to-ground  SetLabelV=off  LabelV=Vabc  Vpu=off  VpuLL=off  CurrentMeasurement=yes  SetLabelI=off  LabelI=Iabc  Ipu=off  Pbase=100e6  Vbase=500e3  OutputType=Complex  PhasorSimulation=on  PSBequivalent=0
      settings: SourceProductName=Simscape Electrical
  A : PMIOPort  Side=Left
  a : PMIOPort  Port=2  Side=Right
  B : PMIOPort  Port=3  Side=Left
  b : PMIOPort  Port=4  Side=Right
  C : PMIOPort  Port=5  Side=Left
  c : PMIOPort  Port=6  Side=Right
  P : Outport
  Q : Outport  Port=2
  wires:
  Three-Phase V-I Measurement/2 -> "Power (3ph, Phasor)"/2
  Three-Phase V-I Measurement/1 -> "Power (3ph, Phasor)"/1
  "Power (3ph, Phasor)"/1 -> P/1
  "Power (3ph, Phasor)"/2 -> Q/1
  connections:
  Three-Phase V-I Measurement/RConn1 -- a/RConn1
  b/RConn1 -- Three-Phase V-I Measurement/RConn2
  A/RConn1 -- Three-Phase V-I Measurement/LConn1
  Three-Phase V-I Measurement/LConn2 -- B/RConn1
  c/RConn1 -- Three-Phase V-I Measurement/RConn3
  C/RConn1 -- Three-Phase V-I Measurement/LConn3

== system tennode_3/DER_Site_1/DER_BESS1/Charge Limits ==
  SOC (%) : Inport
  Pin : Inport  Port=2
  Qin : Inport  Port=3
  Overcharge Check : Subsystem
  Undercharge Check : Subsystem
  Pbatt : Outport
  Qbatt : Outport  Port=2
  wires:
  Overcharge Check/2(Qout) -> Undercharge Check/3(Qin)
  Undercharge Check/1(Pout) -> Pbatt/1  "Pbatt"
  Qin/1 -> Overcharge Check/3(Qin)
  Overcharge Check/1(Pout) -> Undercharge Check/2(Pin)
  Pin/1 -> Overcharge Check/2(Pin)
  Undercharge Check/2(Qout) -> Qbatt/1
  SOC (%)/1 -> Undercharge Check/1(SOC (%)), Overcharge Check/1(SOC (%))

== system tennode_3/DER_Site_1/DER_BESS1/Disable PQ Source if VF Control ==
  Pdes : Inport
  Mode : Inport  Port=2
  Qdes : Inport  Port=3
  Constant : Constant  Value=0
  Constant1 : Constant  Value=0
  Switch2 : Switch  Criteria=u2 > Threshold
  Switch3 : Switch  Criteria=u2 > Threshold
  Pbatt : Outport
  Qbatt : Outport  Port=2
  wires:
  Qdes/1 -> Switch3/1
  Constant/1 -> Switch2/3
  Switch3/1 -> Qbatt/1
  Constant1/1 -> Switch3/3
  Switch2/1 -> Pbatt/1
  Pdes/1 -> Switch2/1
  Mode/1 -> Switch2/2, Switch3/2

== system tennode_3/DER_Site_1/DER_BESS1/Power Measures ==
  EMT : Subsystem  VariantControl=EMT
  Phasor : Subsystem  VariantControl=Phasor
  A : PMIOPort  Side=Left
  a : PMIOPort  Port=2  Side=Right
  B : PMIOPort  Port=3  Side=Left
  b : PMIOPort  Port=4  Side=Right
  C : PMIOPort  Port=5  Side=Left
  c : PMIOPort  Port=6  Side=Right
  P : Outport
  Q : Outport  Port=2

== system tennode_3/DER_Site_1/DER_BESS1/Reactive Power Capability ==
  Pin : Inport
  Qin : Inport  Port=2
  Constant : Constant  Value=Pnom
  Math Function : Math  Operator=square  SaturateOnIntegerOverflow=on
  Math Function1 : Math  Operator=square  SaturateOnIntegerOverflow=on
  Saturation Dynamic : simulink/Discontinuities/Saturation Dynamic  OutMin=[]  OutMax=[]  OutDataTypeStr=Inherit: Same as second input  OutDataType=fixdt(1, 16)  OutScaling=2^-10  DoSatur=off
  Sqrt : Sqrt  SaturateOnIntegerOverflow=on
  Sum : Sum  Inputs=-+|
  Unary Minus : UnaryMinus
  Qout : Outport
  wires:
  Qin/1 -> Saturation Dynamic/2
  Pin/1 -> Math Function1/1
  Saturation Dynamic/1 -> Qout/1
  Unary Minus/1 -> Saturation Dynamic/3
  Sum/1 -> Sqrt/1
  Constant/1 -> Math Function/1
  Math Function/1 -> Sum/2
  Math Function1/1 -> Sum/1
  Sqrt/1 -> Unary Minus/1, Saturation Dynamic/1

== system tennode_3/DER_Site_1/DER_BESS1/Stored Energy Calculation (%) ==
  Pin : Inport
  Qin : Inport  Port=2
  Charge : Gain  Gain=Efficiency/100
  Compare To Zero : simulink/Logic and Bit Operations/Compare To Zero  relop=<=  OutDataTypeStr=boolean
  Constant : Constant  Value=kWh_Rated
  Discharge : Gain  Gain=1/(Efficiency/100)
  Divide : Product  Inputs=*/
  Gain3 : Gain  Gain=1/3600/1e3
  Gain5 : Gain  Gain=-1
  Integrator : Integrator  InitialCondition=(Initial_kWh_pc/100)*kWh_Rated*3600*1e3
  Math Function1 : Math  Operator=square  SaturateOnIntegerOverflow=on
  Math Function2 : Math  Operator=square  SaturateOnIntegerOverflow=on
  Product : Product
  Sign : Signum
  Sqrt : Sqrt  SaturateOnIntegerOverflow=on
  Sum : Sum  Inputs=|++
  Switch1 : Switch  Criteria=u2 ~= 0
  Transfer Fcn : TransferFcn  Denominator=[1 1]
  to % : Gain  Gain=100
  SE% : Outport
  wires:
  Integrator/1 -> Gain3/1
  Compare To Zero/1 -> Switch1/2
  Divide/1 -> to %/1
  Charge/1 -> Switch1/1
  Constant/1 -> Divide/2
  Gain3/1 -> Divide/1
  Switch1/1 -> Gain5/1
  Transfer Fcn/1 -> Compare To Zero/1
  to %/1 -> SE%/1
  Gain5/1 -> Integrator/1
  Discharge/1 -> Switch1/3
  Product/1 -> Charge/1, Discharge/1, Transfer Fcn/1
  Pin/1 -> Sign/1, Math Function1/1
  Qin/1 -> Math Function2/1
  Math Function1/1 -> Sum/1
  Math Function2/1 -> Sum/2
  Sum/1 -> Sqrt/1
  Sqrt/1 -> Product/2
  Sign/1 -> Product/1

== system tennode_3/DER_Site_1/Site Load/Dynamic Load Control ==
  P0 : Inport
  Fcn : Fcn  Expr=sqrt(1/u(1)-1)
  Mux : Mux  Inputs=2
  Product : Product
  Summer1 : Constant  Value=PF
  PQ : Outport
  wires:
  Summer1/1 -> Fcn/1
  Fcn/1 -> Product/2
  P0/1 -> Product/1, Mux/1
  Mux/1 -> PQ/1
  Product/1 -> Mux/2  "Qo"

== system tennode_3/DER_Site_10/DER10_BESS/Charge Limits ==
  SOC (%) : Inport
  Pin : Inport  Port=2
  Qin : Inport  Port=3
  Overcharge Check : Subsystem
  Undercharge Check : Subsystem
  Pbatt : Outport
  Qbatt : Outport  Port=2
  wires:
  Overcharge Check/2(Qout) -> Undercharge Check/3(Qin)
  Undercharge Check/1(Pout) -> Pbatt/1  "Pbatt"
  Qin/1 -> Overcharge Check/3(Qin)
  Overcharge Check/1(Pout) -> Undercharge Check/2(Pin)
  Pin/1 -> Overcharge Check/2(Pin)
  Undercharge Check/2(Qout) -> Qbatt/1
  SOC (%)/1 -> Undercharge Check/1(SOC (%)), Overcharge Check/1(SOC (%))

== system tennode_3/DER_Site_10/DER10_BESS/Disable PQ Source if VF Control ==
  Pdes : Inport
  Mode : Inport  Port=2
  Qdes : Inport  Port=3
  Constant : Constant  Value=0
  Constant1 : Constant  Value=0
  Switch2 : Switch  Criteria=u2 > Threshold
  Switch3 : Switch  Criteria=u2 > Threshold
  Pbatt : Outport
  Qbatt : Outport  Port=2
  wires:
  Qdes/1 -> Switch3/1
  Constant/1 -> Switch2/3
  Switch3/1 -> Qbatt/1
  Constant1/1 -> Switch3/3
  Switch2/1 -> Pbatt/1
  Pdes/1 -> Switch2/1
  Mode/1 -> Switch2/2, Switch3/2

== system tennode_3/DER_Site_10/DER10_BESS/Power Measures ==
  EMT : Subsystem  VariantControl=EMT
  Phasor : Subsystem  VariantControl=Phasor
  A : PMIOPort  Side=Left
  a : PMIOPort  Port=2  Side=Right
  B : PMIOPort  Port=3  Side=Left
  b : PMIOPort  Port=4  Side=Right
  C : PMIOPort  Port=5  Side=Left
  c : PMIOPort  Port=6  Side=Right
  P : Outport
  Q : Outport  Port=2

== system tennode_3/DER_Site_10/DER10_BESS/Reactive Power Capability ==
  Pin : Inport
  Qin : Inport  Port=2
  Constant : Constant  Value=Pnom
  Math Function : Math  Operator=square  SaturateOnIntegerOverflow=on
  Math Function1 : Math  Operator=square  SaturateOnIntegerOverflow=on
  Saturation Dynamic : simulink/Discontinuities/Saturation Dynamic  OutMin=[]  OutMax=[]  OutDataTypeStr=Inherit: Same as second input  OutDataType=fixdt(1, 16)  OutScaling=2^-10  DoSatur=off
  Sqrt : Sqrt  SaturateOnIntegerOverflow=on
  Sum : Sum  Inputs=-+|
  Unary Minus : UnaryMinus
  Qout : Outport
  wires:
  Qin/1 -> Saturation Dynamic/2
  Pin/1 -> Math Function1/1
  Saturation Dynamic/1 -> Qout/1
  Unary Minus/1 -> Saturation Dynamic/3
  Sum/1 -> Sqrt/1
  Constant/1 -> Math Function/1
  Math Function/1 -> Sum/2
  Math Function1/1 -> Sum/1
  Sqrt/1 -> Unary Minus/1, Saturation Dynamic/1

== system tennode_3/DER_Site_10/DER10_BESS/Stored Energy Calculation (%) ==
  Pin : Inport
  Qin : Inport  Port=2
  Charge : Gain  Gain=Efficiency/100
  Compare To Zero : simulink/Logic and Bit Operations/Compare To Zero  relop=<=  OutDataTypeStr=boolean
  Constant : Constant  Value=kWh_Rated
  Discharge : Gain  Gain=1/(Efficiency/100)
  Divide : Product  Inputs=*/
  Gain3 : Gain  Gain=1/3600/1e3
  Gain5 : Gain  Gain=-1
  Integrator : Integrator  InitialCondition=(Initial_kWh_pc/100)*kWh_Rated*3600*1e3
  Math Function1 : Math  Operator=square  SaturateOnIntegerOverflow=on
  Math Function2 : Math  Operator=square  SaturateOnIntegerOverflow=on
  Product : Product
  Sign : Signum
  Sqrt : Sqrt  SaturateOnIntegerOverflow=on
  Sum : Sum  Inputs=|++
  Switch1 : Switch  Criteria=u2 ~= 0
  Transfer Fcn : TransferFcn  Denominator=[1 1]
  to % : Gain  Gain=100
  SE% : Outport
  wires:
  Integrator/1 -> Gain3/1
  Compare To Zero/1 -> Switch1/2
  Divide/1 -> to %/1
  Charge/1 -> Switch1/1
  Constant/1 -> Divide/2
  Gain3/1 -> Divide/1
  Switch1/1 -> Gain5/1
  Transfer Fcn/1 -> Compare To Zero/1
  to %/1 -> SE%/1
  Gain5/1 -> Integrator/1
  Discharge/1 -> Switch1/3
  Product/1 -> Charge/1, Discharge/1, Transfer Fcn/1
  Pin/1 -> Sign/1, Math Function1/1
  Qin/1 -> Math Function2/1
  Math Function1/1 -> Sum/1
  Math Function2/1 -> Sum/2
  Sum/1 -> Sqrt/1
  Sqrt/1 -> Product/2
  Sign/1 -> Product/1

== system tennode_3/DER_Site_10/Site Load/Dynamic Load Control ==
  P0 : Inport
  Fcn : Fcn  Expr=sqrt(1/u(1)-1)
  Mux : Mux  Inputs=2
  Product : Product
  Summer1 : Constant  Value=PF
  PQ : Outport
  wires:
  Summer1/1 -> Fcn/1
  Fcn/1 -> Product/2
  P0/1 -> Product/1, Mux/1
  Mux/1 -> PQ/1
  Product/1 -> Mux/2  "Qo"

== system tennode_3/DER_Site_2/DER2_BESS/Charge Limits ==
  SOC (%) : Inport
  Pin : Inport  Port=2
  Qin : Inport  Port=3
  Overcharge Check : Subsystem
  Undercharge Check : Subsystem
  Pbatt : Outport
  Qbatt : Outport  Port=2
  wires:
  Overcharge Check/2(Qout) -> Undercharge Check/3(Qin)
  Undercharge Check/1(Pout) -> Pbatt/1  "Pbatt"
  Qin/1 -> Overcharge Check/3(Qin)
  Overcharge Check/1(Pout) -> Undercharge Check/2(Pin)
  Pin/1 -> Overcharge Check/2(Pin)
  Undercharge Check/2(Qout) -> Qbatt/1
  SOC (%)/1 -> Undercharge Check/1(SOC (%)), Overcharge Check/1(SOC (%))

== system tennode_3/DER_Site_2/DER2_BESS/Disable PQ Source if VF Control ==
  Pdes : Inport
  Mode : Inport  Port=2
  Qdes : Inport  Port=3
  Constant : Constant  Value=0
  Constant1 : Constant  Value=0
  Switch2 : Switch  Criteria=u2 > Threshold
  Switch3 : Switch  Criteria=u2 > Threshold
  Pbatt : Outport
  Qbatt : Outport  Port=2
  wires:
  Qdes/1 -> Switch3/1
  Constant/1 -> Switch2/3
  Switch3/1 -> Qbatt/1
  Constant1/1 -> Switch3/3
  Switch2/1 -> Pbatt/1
  Pdes/1 -> Switch2/1
  Mode/1 -> Switch2/2, Switch3/2

== system tennode_3/DER_Site_2/DER2_BESS/Power Measures ==
  EMT : Subsystem  VariantControl=EMT
  Phasor : Subsystem  VariantControl=Phasor
  A : PMIOPort  Side=Left
  a : PMIOPort  Port=2  Side=Right
  B : PMIOPort  Port=3  Side=Left
  b : PMIOPort  Port=4  Side=Right
  C : PMIOPort  Port=5  Side=Left
  c : PMIOPort  Port=6  Side=Right
  P : Outport
  Q : Outport  Port=2

== system tennode_3/DER_Site_2/DER2_BESS/Reactive Power Capability ==
  Pin : Inport
  Qin : Inport  Port=2
  Constant : Constant  Value=Pnom
  Math Function : Math  Operator=square  SaturateOnIntegerOverflow=on
  Math Function1 : Math  Operator=square  SaturateOnIntegerOverflow=on
  Saturation Dynamic : simulink/Discontinuities/Saturation Dynamic  OutMin=[]  OutMax=[]  OutDataTypeStr=Inherit: Same as second input  OutDataType=fixdt(1, 16)  OutScaling=2^-10  DoSatur=off
  Sqrt : Sqrt  SaturateOnIntegerOverflow=on
  Sum : Sum  Inputs=-+|
  Unary Minus : UnaryMinus
  Qout : Outport
  wires:
  Qin/1 -> Saturation Dynamic/2
  Pin/1 -> Math Function1/1
  Saturation Dynamic/1 -> Qout/1
  Unary Minus/1 -> Saturation Dynamic/3
  Sum/1 -> Sqrt/1
  Constant/1 -> Math Function/1
  Math Function/1 -> Sum/2
  Math Function1/1 -> Sum/1
  Sqrt/1 -> Unary Minus/1, Saturation Dynamic/1

== system tennode_3/DER_Site_2/DER2_BESS/Stored Energy Calculation (%) ==
  Pin : Inport
  Qin : Inport  Port=2
  Charge : Gain  Gain=Efficiency/100
  Compare To Zero : simulink/Logic and Bit Operations/Compare To Zero  relop=<=  OutDataTypeStr=boolean
  Constant : Constant  Value=kWh_Rated
  Discharge : Gain  Gain=1/(Efficiency/100)
  Divide : Product  Inputs=*/
  Gain3 : Gain  Gain=1/3600/1e3
  Gain5 : Gain  Gain=-1
  Integrator : Integrator  InitialCondition=(Initial_kWh_pc/100)*kWh_Rated*3600*1e3
  Math Function1 : Math  Operator=square  SaturateOnIntegerOverflow=on
  Math Function2 : Math  Operator=square  SaturateOnIntegerOverflow=on
  Product : Product
  Sign : Signum
  Sqrt : Sqrt  SaturateOnIntegerOverflow=on
  Sum : Sum  Inputs=|++
  Switch1 : Switch  Criteria=u2 ~= 0
  Transfer Fcn : TransferFcn  Denominator=[1 1]
  to % : Gain  Gain=100
  SE% : Outport
  wires:
  Integrator/1 -> Gain3/1
  Compare To Zero/1 -> Switch1/2
  Divide/1 -> to %/1
  Charge/1 -> Switch1/1
  Constant/1 -> Divide/2
  Gain3/1 -> Divide/1
  Switch1/1 -> Gain5/1
  Transfer Fcn/1 -> Compare To Zero/1
  to %/1 -> SE%/1
  Gain5/1 -> Integrator/1
  Discharge/1 -> Switch1/3
  Product/1 -> Charge/1, Discharge/1, Transfer Fcn/1
  Pin/1 -> Sign/1, Math Function1/1
  Qin/1 -> Math Function2/1
  Math Function1/1 -> Sum/1
  Math Function2/1 -> Sum/2
  Sum/1 -> Sqrt/1
  Sqrt/1 -> Product/2
  Sign/1 -> Product/1

== system tennode_3/DER_Site_2/Site Load/Dynamic Load Control ==
  P0 : Inport
  Fcn : Fcn  Expr=sqrt(1/u(1)-1)
  Mux : Mux  Inputs=2
  Product : Product
  Summer1 : Constant  Value=PF
  PQ : Outport
  wires:
  Summer1/1 -> Fcn/1
  Fcn/1 -> Product/2
  P0/1 -> Product/1, Mux/1
  Mux/1 -> PQ/1
  Product/1 -> Mux/2  "Qo"

== system tennode_3/DER_Site_3/DER3_BESS/Charge Limits ==
  SOC (%) : Inport
  Pin : Inport  Port=2
  Qin : Inport  Port=3
  Overcharge Check : Subsystem
  Undercharge Check : Subsystem
  Pbatt : Outport
  Qbatt : Outport  Port=2
  wires:
  Overcharge Check/2(Qout) -> Undercharge Check/3(Qin)
  Undercharge Check/1(Pout) -> Pbatt/1  "Pbatt"
  Qin/1 -> Overcharge Check/3(Qin)
  Overcharge Check/1(Pout) -> Undercharge Check/2(Pin)
  Pin/1 -> Overcharge Check/2(Pin)
  Undercharge Check/2(Qout) -> Qbatt/1
  SOC (%)/1 -> Undercharge Check/1(SOC (%)), Overcharge Check/1(SOC (%))

== system tennode_3/DER_Site_3/DER3_BESS/Disable PQ Source if VF Control ==
  Pdes : Inport
  Mode : Inport  Port=2
  Qdes : Inport  Port=3
  Constant : Constant  Value=0
  Constant1 : Constant  Value=0
  Switch2 : Switch  Criteria=u2 > Threshold
  Switch3 : Switch  Criteria=u2 > Threshold
  Pbatt : Outport
  Qbatt : Outport  Port=2
  wires:
  Qdes/1 -> Switch3/1
  Constant/1 -> Switch2/3
  Switch3/1 -> Qbatt/1
  Constant1/1 -> Switch3/3
  Switch2/1 -> Pbatt/1
  Pdes/1 -> Switch2/1
  Mode/1 -> Switch2/2, Switch3/2

== system tennode_3/DER_Site_3/DER3_BESS/Power Measures ==
  EMT : Subsystem  VariantControl=EMT
  Phasor : Subsystem  VariantControl=Phasor
  A : PMIOPort  Side=Left
  a : PMIOPort  Port=2  Side=Right
  B : PMIOPort  Port=3  Side=Left
  b : PMIOPort  Port=4  Side=Right
  C : PMIOPort  Port=5  Side=Left
  c : PMIOPort  Port=6  Side=Right
  P : Outport
  Q : Outport  Port=2

== system tennode_3/DER_Site_3/DER3_BESS/Reactive Power Capability ==
  Pin : Inport
  Qin : Inport  Port=2
  Constant : Constant  Value=Pnom
  Math Function : Math  Operator=square  SaturateOnIntegerOverflow=on
  Math Function1 : Math  Operator=square  SaturateOnIntegerOverflow=on
  Saturation Dynamic : simulink/Discontinuities/Saturation Dynamic  OutMin=[]  OutMax=[]  OutDataTypeStr=Inherit: Same as second input  OutDataType=fixdt(1, 16)  OutScaling=2^-10  DoSatur=off
  Sqrt : Sqrt  SaturateOnIntegerOverflow=on
  Sum : Sum  Inputs=-+|
  Unary Minus : UnaryMinus
  Qout : Outport
  wires:
  Qin/1 -> Saturation Dynamic/2
  Pin/1 -> Math Function1/1
  Saturation Dynamic/1 -> Qout/1
  Unary Minus/1 -> Saturation Dynamic/3
  Sum/1 -> Sqrt/1
  Constant/1 -> Math Function/1
  Math Function/1 -> Sum/2
  Math Function1/1 -> Sum/1
  Sqrt/1 -> Unary Minus/1, Saturation Dynamic/1
